simulink model "sim_Ex5"  (R2022b)
settings: Solver=VariableStepAuto  StartTime=0.0  StopTime=10.0  FixedStep=1e-3  MaxStep=1e-4  RelTol=1e-4
values from neighbouring files (symbols this model uses):
  L = LengthArray(i)    [sim_Ex5_script.m]
settings Model: Creator=MAAM  LastModifiedBy=MAAM

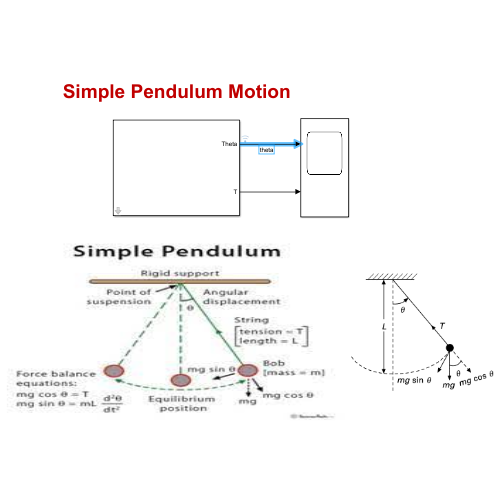
[thumbnail: Simulink's stored preview of the top-level diagram]
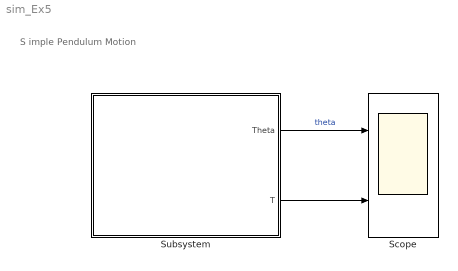
== system sim_Ex5 ==
  note: S imple Pendulum Motion
  Scope : Scope  NumInputPorts=2
  Subsystem : Subsystem  mask{theta0=60*pi/180, L=L, m=1, g=9.81, Damp=off, b=0.25}
      mask prompts: L "Length (m) L"; m "Mass (Kg) m"; g "Grafity Acc (m/s^2) g"; Damp "apply Damping Coefficient"; b "Damping Coefficient (Kg/s) b"
      mask init:
      | % Check the value of the checkbox
      | if isequal(Damp, 1)
      |     % Make the parameter visible
      |     set_param(gcb, 'MaskVisibilities', {'on', 'on', 'on', 'on', 'on', 'on'});
      | else
      |     % Hide the parameter
      |     set_param(gcb, 'MaskVisibilities', {'on', 'on', 'on', 'on', 'on', 'off'});
      | end
  wires:
  Subsystem/1(Theta) -> Scope/1  "theta"
  Subsystem/2(T) -> Scope/2

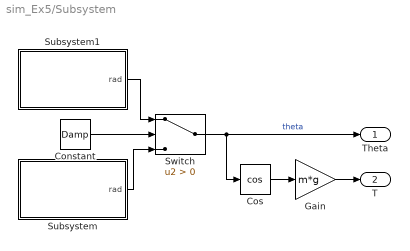
== system sim_Ex5/Subsystem ==
  Constant : Constant  Value=Damp
  Cos : Trigonometry  Operator=cos
  Gain : Gain  Gain=m*g
  Subsystem : Subsystem
  Subsystem1 : Subsystem
  Switch : Switch  Criteria=u2 > Threshold  SaturateOnIntegerOverflow=off  InputSameDT=off
  Theta : Outport
  T : Outport  Port=2
  wires:
  Constant/1 -> Switch/2
  Switch/1 -> Cos/1, Theta/1  "theta"
  Subsystem1/1(rad) -> Switch/1
  Cos/1 -> Gain/1
  Gain/1 -> T/1
  Subsystem/1(rad) -> Switch/3

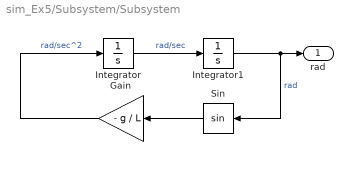
== system sim_Ex5/Subsystem/Subsystem ==
  Gain : Gain  Gain=- g / L
  Integrator : Integrator
  Integrator1 : Integrator  InitialCondition=theta0
  Sin : Trigonometry
  rad : Outport
  wires:
  Integrator1/1 -> Sin/1, rad/1  "rad"
  Gain/1 -> Integrator/1  "rad/sec^2"
  Integrator/1 -> Integrator1/1  "rad/sec"
  Sin/1 -> Gain/1

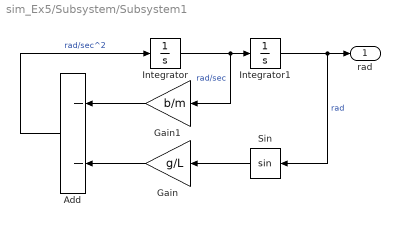
== system sim_Ex5/Subsystem/Subsystem1 ==
  Add : Sum  Inputs=--
  Gain : Gain  Gain=g/L
  Gain1 : Gain  Gain=b/m
  Integrator : Integrator
  Integrator1 : Integrator  InitialCondition=theta0
  Sin : Trigonometry
  rad : Outport
  wires:
  Sin/1 -> Gain/1
  Integrator/1 -> Gain1/1, Integrator1/1  "rad/sec"
  Add/1 -> Integrator/1  "rad/sec^2"
  Integrator1/1 -> rad/1, Sin/1  "rad"
  Gain/1 -> Add/2
  Gain1/1 -> Add/1
